simulink model "PImasDdf"  (R2016a)
settings: Solver=FixedStepDiscrete  StartTime=0.0  StopTime=30
undefined symbols (not defined in the file or in its folder): DiscIntNeverNeededParam
libraries: simulink x2, fuzblock x1
settings Model: Creator=PC  LastModifiedBy=PC
settings SolverCC: MaxConsecutiveZCs=10000  SolverJacobianMethodControl=FullAnalytical  ZeroCrossControl=DisableAll  ZeroCrossAlgorithm=Adaptive  AutoInsertRateTranBlk=on
settings DataIOCC: LimitDataPoints=on  SaveOutput=off  SaveTime=off  Refine=10
settings OptimizationCC: ExpressionDepthLimit=2147483647  LifeSpan=1
settings DebuggingCC: UnderspecifiedInitializationDetection=Classic  MergeDetectMultiDrivingBlocksExec=none  FcnCallInpInsideContextMsg=EnableAllAsWarning  AllowSymbolicDim=off  StateNameClashWarn=warning
settings GRTTargetCC: CombineOutputUpdateFcns=off  GRTInterface=on

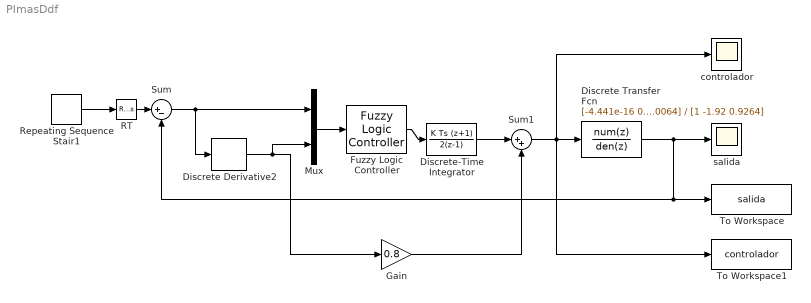
== system PImasDdf ==
  Discrete Transfer Fcn : DiscreteTransferFcn  Numerator=[-4.441e-16 0.0064]  Denominator=[1 -1.92 0.9264]  SampleTime=0.08
  Discrete Derivative2 : simulink/Discrete/Discrete Derivative  gainval=1.0  ICPrevScaledInput=0.0  OutMin=[]  OutMax=[]  OutDataType=fixdt(1, 16)  OutScaling=2^-10  DoSatur=off
  Discrete-Time Integrator : DiscreteIntegrator  IntegratorMethod=Integration: Trapezoidal  InitialConditionSetting=State (most efficient)  SampleTime=0.08  ICPrevOutput=DiscIntNeverNeededParam  ICPrevScaledInput=DiscIntNeverNeededParam
  Fuzzy Logic Controller : fuzblock/Fuzzy Logic  Controller  fis='PI.fis'
  Gain : Gain  Gain=0.8
  Mux : Mux  Inputs=2
  RT : RateTransition  Deterministic=off  OutPortSampleTime=0.08
  Repeating Sequence Stair1 : simulink/Sources/Repeating Sequence Stair  OutValues=[0 0 1 1 1 1 1 1 0.5 0.5 0.5 0.5 0.5 0.5 0.5 0.5 0.25 0.25 0.25 0.25 0.25 0.25 0.25 1 1 1 1 1 1 1 1 1 1 1 1 1].'  tsamp=1  OutMin=[]  OutMax=[]  OutDataTypeStr=double  OutputDataTypeScalingMode=double  OutDataType=fixdt(0,8)  ConRadixGroup=Best Precision: Vector-wise  OutScaling=2^-12
  Sum : Sum  Inputs=|+-
  Sum1 : Sum  Inputs=|++
  To Workspace : ToWorkspace  VariableName=salida  SaveFormat=Timeseries  SampleTime=-1
  To Workspace1 : ToWorkspace  VariableName=controlador  SaveFormat=Timeseries  SampleTime=-1
  controlador : Scope
  "salida " : Scope
  wires:
  Discrete Transfer Fcn/1 -> "salida "/1, Sum/2, To Workspace/1
  Fuzzy Logic Controller/1 -> Discrete-Time Integrator/1
  Mux/1 -> Fuzzy Logic Controller/1
  Sum/1 -> Mux/1, Discrete Derivative2/1
  Gain/1 -> Sum1/2
  Repeating Sequence Stair1/1 -> RT/1
  Discrete Derivative2/1 -> Mux/2, Gain/1
  Discrete-Time Integrator/1 -> Sum1/1
  Sum1/1 -> Discrete Transfer Fcn/1, To Workspace1/1, controlador/1
  RT/1 -> Sum/1
